simulink model "HeldBeneathReset"  (R2015a)
settings: Solver=FixedStepDiscrete  SolverMode=SingleTasking  StartTime=0.0  StopTime=100  FixedStep=1  RelTol=1e-3
settings Model: CovMetricSettings=dwe  CovHtmlReporting=off  covSaveCumulativeToWorkspaceVar=off  CovSaveSingleToWorkspaceVar=off  CovExternalEMLEnable=on  Creator=hbourbou  LastModifiedBy=hbourbou
settings DataIOCC: LimitDataPoints=off  SaveFormat=Dataset
settings DebuggingCC: SFUnexpectedBacktrackingDiag=error  SFNoUnconditionalDefaultTransitionDiag=error
settings HardwareCC: ProdBitPerPointer=64  ProdLargestAtomicFloat=Float  ProdIntDivRoundTo=Zero  ProdEndianess=LittleEndian  ProdHWDeviceType=Specified
settings ModelReferenceCC: PropagateSignalLabelsOutOfModel=on
settings GRTTargetCC: TargetLangStandard=C99 (ISO)  GeneratePreprocessorConditionals=Use local settings

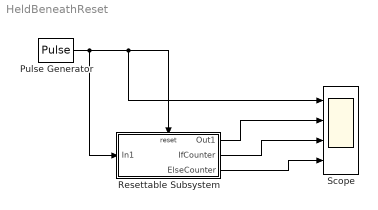
== system HeldBeneathReset ==
  Pulse Generator : DiscretePulseGenerator  Period=4  PulseWidth=2  SampleTime=-1
      settings: AttributesFormatString=Period: %<period>\nDuty cycle: %<pulsewidth>%
  Resettable Subsystem : Subsystem  TreatAsAtomicUnit=on
  Scope : Scope  NumInputPorts=4
      settings: TimeRange=auto  MaxDataPoints=5000  SaveToWorkspace=off  SaveName=ScopeData  YMin=-0.125~0.875~-5.25~-6.25  YMax=1.125~2.125~57.25~56.25  SampleTime=-1
  wires:
  Pulse Generator/1 -> Resettable Subsystem/1(In1), Scope/1, Resettable Subsystem/Reset
  Resettable Subsystem/1(Out1) -> Scope/2
  Resettable Subsystem/2(IfCounter) -> Scope/3
  Resettable Subsystem/3(ElseCounter) -> Scope/4

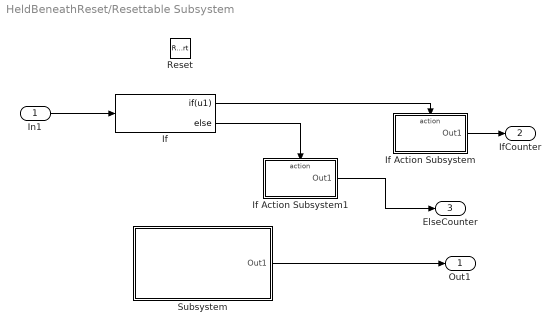
== system HeldBeneathReset/Resettable Subsystem ==
  In1 : Inport
  Reset : ResetPort  DisableCoverage=on  ResetTriggerType=either
  If : If  IfExpression=u1
  If Action Subsystem : Subsystem  TreatAsAtomicUnit=on
  If Action Subsystem1 : Subsystem  TreatAsAtomicUnit=on
  Subsystem : Subsystem  TreatAsAtomicUnit=on
  Out1 : Outport
  IfCounter : Outport  Port=2
  ElseCounter : Outport  Port=3
  wires:
  In1/1 -> If/1
  If/1 -> If Action Subsystem/Action
  If/2 -> If Action Subsystem1/Action
  If Action Subsystem/1(Out1) -> IfCounter/1
  If Action Subsystem1/1(Out1) -> ElseCounter/1
  Subsystem/1(Out1) -> Out1/1

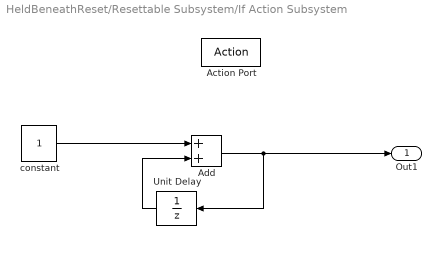
== system HeldBeneathReset/Resettable Subsystem/If Action Subsystem ==
  Action Port : ActionPort  ActionType=then
  Add : Sum
  Unit Delay : UnitDelay  SampleTime=-1
  constant : Constant
  Out1 : Outport  InitialOutput=0
  wires:
  Add/1 -> Unit Delay/1, Out1/1
  constant/1 -> Add/1
  Unit Delay/1 -> Add/2

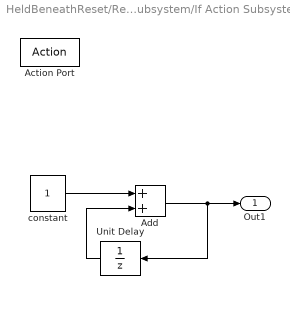
== system HeldBeneathReset/Resettable Subsystem/If Action Subsystem1 ==
  Action Port : ActionPort  ActionType=else
  Add : Sum
  Unit Delay : UnitDelay  SampleTime=-1
  constant : Constant
  Out1 : Outport
  wires:
  Add/1 -> Unit Delay/1, Out1/1
  constant/1 -> Add/1
  Unit Delay/1 -> Add/2

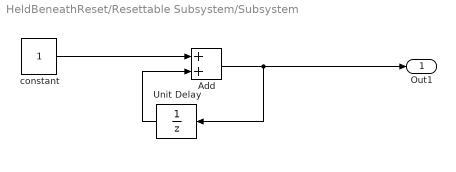
== system HeldBeneathReset/Resettable Subsystem/Subsystem ==
  Add : Sum
  Unit Delay : UnitDelay  SampleTime=-1
  constant : Constant
  Out1 : Outport
  wires:
  constant/1 -> Add/1
  Add/1 -> Out1/1, Unit Delay/1
  Unit Delay/1 -> Add/2
